simulink model "BCM_C1A_CombiSwitch_9"  (R2018b)
settings: Solver=FixedStepDiscrete  StartTime=0.0  StopTime=10.0  FixedStep=0.01  RelTol=1e-3
undefined symbols (not defined in the file or in its folder): TYP_CSW_INT_POSITION, TYP_EXT_LIGHTS, TYP_FRONT_WIPER, TYP_LIGHTING_CSW, TYP_REAR_WIPER, TYP_VEHICLE_STATE
libraries: Renault_Library x80, library_BCM x2
(part 2 of 3)

== system BCM_C1A_CombiSwitch_9/CombiSwitch/COMBINATION_SWITCH_FNS/EXTERNAL_LIGHTS_MANAGEMENT ==
  R_EXT_LIGHTS : Inport  OutDataTypeStr=Enum: TYP_EXT_LIGHTS
      settings: AttributesFormatString=Type : %<OutDataTypeStr>
  COMBI_SW_FAILURE_TFAIL : Inport  Port=2  OutDataTypeStr=boolean
      settings: AttributesFormatString=Type : %<OutDataTypeStr>
  LIGHTING_CSW_FAILURE_MODE : Inport  Port=3  OutDataTypeStr=boolean
      settings: AttributesFormatString=Type : %<OutDataTypeStr>
  CSW_IN_FAILURE_MODE : Inport  Port=4  OutDataTypeStr=boolean
      settings: AttributesFormatString=Type : %<OutDataTypeStr>
  IN_DRIVING_CYCLE : Inport  Port=5  OutDataTypeStr=boolean
      settings: AttributesFormatString=Type : %<OutDataTypeStr>
  LIGHTING_CSW_CONFIGURATION_CF : Inport  Port=6  OutDataTypeStr=Enum: TYP_LIGHTING_CSW
      settings: AttributesFormatString=Type : %<OutDataTypeStr>
  Constant1 : Constant  Value=TYP_LIGHTING_CSW.LIGHTING_CSW_WORLD_WITHOUT_ALS  OutDataTypeStr=Enum: TYP_LIGHTING_CSW  SampleTime=-1
  Constant2 : Constant  Value=TYP_LIGHTING_CSW.LIGHTING_CSW_WORLD_WITH_ALS  OutDataTypeStr=Enum: TYP_LIGHTING_CSW  SampleTime=-1
  Constant4 : Constant  Value=TYP_LIGHTING_CSW.LIGHTING_CSW_FOR_EUROPE  OutDataTypeStr=Enum: TYP_LIGHTING_CSW  SampleTime=-1
  Constant5 : Constant  Value=TYP_LIGHTING_CSW.LIGHTING_CSW_FOR_EUROPE  OutDataTypeStr=Enum: TYP_LIGHTING_CSW  SampleTime=-1
  LogicalOperator : Logic  Operator=OR  OutDataTypeStr=boolean
  R_LIGHT_SW_EUROPE : Subsystem  TreatAsAtomicUnit=on
      settings: RTWSystemCode=Inline
  R_LIGHT_SW_WORLD : Subsystem  TreatAsAtomicUnit=on
      settings: RTWSystemCode=Inline
  RelationalOperator{,1..3} (4 alike) : RelationalOperator  Operator===  OutDataTypeStr=boolean  RndMeth=Nearest  InputSameDT=on
  Switch : Switch  Criteria=u2 ~= 0  RndMeth=Zero  InputSameDT=on
      settings: AttributesFormatString=Criteria=%<Criteria>
  R_LIGHTS_SW : Outport  OutDataTypeStr=Enum: TYP_EXT_LIGHTS
      settings: AttributesFormatString=Type : %<OutDataTypeStr>\nInit :%<InitialOutput>
  wires:
  [IN_DRIVING_CYCLE] -> R_LIGHT_SW_WORLD/5(IN_DRIVING_CYCLE)
  [LIGHTING_CSW_FAILURE_MODE] -> R_LIGHT_SW_WORLD/3(LIGHTING_CSW_FAILURE_MODE)
  [COMBI_SW_FAILURE_TFAIL] -> R_LIGHT_SW_WORLD/2(COMBI_SW_FAILURE_TFAIL)
  [CSW_IN_FAILURE_MODE] -> R_LIGHT_SW_WORLD/4(CSW_IN_FAILURE_MODE)
  [R_EXT_LIGHTS] -> R_LIGHT_SW_WORLD/1(R_EXT_LIGHTS)
  LIGHTING_CSW_CONFIGURATION_CF/1 -> [LIGHTING_CSW_CONFIGURATION_CF]
  R_EXT_LIGHTS/1 -> [R_EXT_LIGHTS]
  IN_DRIVING_CYCLE/1 -> [IN_DRIVING_CYCLE]
  CSW_IN_FAILURE_MODE/1 -> [CSW_IN_FAILURE_MODE]
  LIGHTING_CSW_FAILURE_MODE/1 -> [LIGHTING_CSW_FAILURE_MODE]
  COMBI_SW_FAILURE_TFAIL/1 -> [COMBI_SW_FAILURE_TFAIL]
  [IN_DRIVING_CYCLE] -> R_LIGHT_SW_EUROPE/5(IN_DRIVING_CYCLE)
  [LIGHTING_CSW_FAILURE_MODE] -> R_LIGHT_SW_EUROPE/3(LIGHTING_CSW_FAILURE_MODE)
  [COMBI_SW_FAILURE_TFAIL] -> R_LIGHT_SW_EUROPE/2(COMBI_SW_FAILURE_TFAIL)
  [CSW_IN_FAILURE_MODE] -> R_LIGHT_SW_EUROPE/4(CSW_IN_FAILURE_MODE)
  [R_EXT_LIGHTS] -> R_LIGHT_SW_EUROPE/1(R_EXT_LIGHTS)
  RelationalOperator1/1 -> R_LIGHT_SW_EUROPE/Enable
  [LIGHTING_CSW_CONFIGURATION_CF] -> RelationalOperator1/1
  [LIGHTING_CSW_CONFIGURATION_CF] -> RelationalOperator/1
  Constant2/1 -> RelationalOperator/2
  Constant1/1 -> RelationalOperator2/2
  [LIGHTING_CSW_CONFIGURATION_CF] -> RelationalOperator2/1
  RelationalOperator/1 -> LogicalOperator/1
  RelationalOperator2/1 -> LogicalOperator/2
  LogicalOperator/1 -> R_LIGHT_SW_WORLD/Enable
  [LIGHTING_CSW_CONFIGURATION_CF] -> RelationalOperator3/1
  Constant5/1 -> RelationalOperator3/2
  RelationalOperator3/1 -> Switch/2
  Switch/1 -> R_LIGHTS_SW/1
  R_LIGHT_SW_EUROPE/1(R_LIGHTS_SW_EUROPE) -> Switch/1
  R_LIGHT_SW_WORLD/1(R_LIGHTS_SW_WORLD) -> Switch/3
  Constant4/1 -> RelationalOperator1/2

== system BCM_C1A_CombiSwitch_9/CombiSwitch/COMBINATION_SWITCH_FNS/FLASHERS_MANAGEMENT ==
  R_FLASH_LEFT : Inport  OutDataTypeStr=boolean
      settings: AttributesFormatString=Type : %<OutDataTypeStr>
  R_FLASH_RIGHT : Inport  Port=2  OutDataTypeStr=boolean
      settings: AttributesFormatString=Type : %<OutDataTypeStr>
  R_FLASH_LEFT_SW : Outport  OutDataTypeStr=boolean
      settings: AttributesFormatString=Type : %<OutDataTypeStr>\nInit :%<InitialOutput>
  R_FLASH_RIGHT_SW : Outport  Port=2  OutDataTypeStr=boolean
      settings: AttributesFormatString=Type : %<OutDataTypeStr>\nInit :%<InitialOutput>
  wires:
  R_FLASH_RIGHT/1 -> R_FLASH_RIGHT_SW/1
  R_FLASH_LEFT/1 -> R_FLASH_LEFT_SW/1

== system BCM_C1A_CombiSwitch_9/CombiSwitch/COMBINATION_SWITCH_FNS/FRONT_FOG_MANAGEMENT ==
  R_FR_FOG : Inport  OutDataTypeStr=boolean
      settings: AttributesFormatString=Type : %<OutDataTypeStr>
  COMBI_SW_FAILURE_TFAIL : Inport  Port=2  OutDataTypeStr=boolean
      settings: AttributesFormatString=Type : %<OutDataTypeStr>
  LogicalOperator : Logic  OutDataTypeStr=boolean
  LogicalOperator1 : Logic  Operator=NOT  Inputs=1  OutDataTypeStr=boolean
  R_FR_FOG_SW : Outport  OutDataTypeStr=boolean
      settings: AttributesFormatString=Type : %<OutDataTypeStr>\nInit :%<InitialOutput>
  wires:
  R_FR_FOG/1 -> LogicalOperator/1
  LogicalOperator1/1 -> LogicalOperator/2
  LogicalOperator/1 -> R_FR_FOG_SW/1
  COMBI_SW_FAILURE_TFAIL/1 -> LogicalOperator1/1

== system BCM_C1A_CombiSwitch_9/CombiSwitch/COMBINATION_SWITCH_FNS/FRONT_WIPER_MANAGEMENT ==
  R_FRONT_WIPER : Inport  OutDataTypeStr=Enum: TYP_FRONT_WIPER
      settings: AttributesFormatString=Type : %<OutDataTypeStr>
  R_INT_TIME : Inport  Port=2  OutDataTypeStr=Enum: TYP_CSW_INT_POSITION
      settings: AttributesFormatString=Type : %<OutDataTypeStr>
  CSW_IN_FAILURE_MODE : Inport  Port=3  OutDataTypeStr=boolean
      settings: AttributesFormatString=Type : %<OutDataTypeStr>
  COMBI_SW_FAILURE_TFAIL : Inport  Port=4  OutDataTypeStr=boolean
      settings: AttributesFormatString=Type : %<OutDataTypeStr>
  IN_DRIVING_CYCLE : Inport  Port=5  OutDataTypeStr=boolean
      settings: AttributesFormatString=Type : %<OutDataTypeStr>
  Constant1 : Constant  Value=TYP_FRONT_WIPER.CSW_OFF_FW  OutDataTypeStr=Enum: TYP_FRONT_WIPER  SampleTime=-1
  LogicalOperator2 : Logic  Operator=OR  OutDataTypeStr=boolean
  LogicalOperator3 : Logic  OutDataTypeStr=boolean
  LogicalOperator4 : Logic  Operator=NOT  Inputs=1  OutDataTypeStr=boolean
  LogicalOperator6 : Logic  OutDataTypeStr=boolean
  RSA_DetectChange_v01_04 : Renault_Library/Complex blocks/Logic & Bit Operations/RSA_DetectChange_v01_04  Tag=[LIB]  chkini=on  vinit=false
      settings: AttributesFormatString=%<MaskType> : Ver : 01.04\nCompare the Input with Initial Value = %<chkini>\nInitial Value : = %<vinit>
  RSA_DetectChange_v01_1 : Renault_Library/Complex blocks/Logic & Bit Operations/RSA_DetectChange_v01_04  Tag=[LIB]  chkini=on  vinit=false
      settings: AttributesFormatString=%<MaskType> : Ver : 01.04\nCompare the Input with Initial Value = %<chkini>\nInitial Value : = %<vinit>
  Switch1 : Switch  Criteria=u2 ~= 0  RndMeth=Zero  InputSameDT=on
      settings: AttributesFormatString=Criteria=%<Criteria>
  Switch4 : Switch  Criteria=u2 ~= 0  RndMeth=Zero  InputSameDT=on
      settings: AttributesFormatString=Criteria=%<Criteria>
  Switch6 : Switch  Criteria=u2 ~= 0  RndMeth=Zero  InputSameDT=on
      settings: AttributesFormatString=Criteria=%<Criteria>
  UnitDelay : UnitDelay  InitialCondition=TYP_FRONT_WIPER.CSW_OFF_FW  SampleTime=-1
      settings: AttributesFormatString=IC = %<X0>
  UnitDelay2 : UnitDelay  InitialCondition=TYP_CSW_INT_POSITION.CSW_INTERMITTENT_POSITION_1  SampleTime=-1
      settings: AttributesFormatString=IC = %<X0>
  R_FR_WIPER_SW : Outport  OutDataTypeStr=Enum: TYP_FRONT_WIPER
      settings: AttributesFormatString=Type : %<OutDataTypeStr>\nInit :%<InitialOutput>
  R_INT_SW : Outport  Port=2  OutDataTypeStr=Enum: TYP_CSW_INT_POSITION
      settings: AttributesFormatString=Type : %<OutDataTypeStr>\nInit :%<InitialOutput>
  wires:
  [R_INT_TIME] -> Switch6/3
  R_INT_TIME/1 -> [R_INT_TIME]
  [R_FRONT_WIPER] -> Switch4/3
  R_FRONT_WIPER/1 -> [R_FRONT_WIPER]
  RSA_DetectChange_v01_1/1 -> LogicalOperator2/2
  RSA_DetectChange_v01_04/1 -> LogicalOperator2/1
  LogicalOperator4/1 -> LogicalOperator6/2
  LogicalOperator3/1 -> Switch1/2
  LogicalOperator6/1 -> LogicalOperator3/2
  LogicalOperator2/1 -> LogicalOperator3/1
  [IN_DRIVING_CYCLE] -> RSA_DetectChange_v01_1/1
  [CSW_IN_FAILURE_MODE] -> RSA_DetectChange_v01_04/1
  UnitDelay2/1 -> Switch6/1
  [COMBI_SW_FAILURE_TFAIL] -> Switch6/2
  [R_INT_SW] -> UnitDelay2/1
  Switch1/1 -> Switch4/1
  [COMBI_SW_FAILURE_TFAIL] -> Switch4/2
  Switch6/1 -> R_INT_SW/1, [R_INT_SW]
  [IN_DRIVING_CYCLE] -> LogicalOperator4/1
  UnitDelay/1 -> Switch1/3
  [R_FR_WIPER_SW] -> UnitDelay/1
  Constant1/1 -> Switch1/1
  Switch4/1 -> [R_FR_WIPER_SW], R_FR_WIPER_SW/1
  [CSW_IN_FAILURE_MODE] -> LogicalOperator6/1
  CSW_IN_FAILURE_MODE/1 -> [CSW_IN_FAILURE_MODE]
  COMBI_SW_FAILURE_TFAIL/1 -> [COMBI_SW_FAILURE_TFAIL]
  IN_DRIVING_CYCLE/1 -> [IN_DRIVING_CYCLE]

== system BCM_C1A_CombiSwitch_9/CombiSwitch/COMBINATION_SWITCH_FNS/HIGH_BEAM_MANAGEMENT ==
  R_HIGH_BEAM : Inport  OutDataTypeStr=boolean
      settings: AttributesFormatString=Type : %<OutDataTypeStr>
  LIGHTING_CSW_FAILURE_MODE : Inport  Port=2  OutDataTypeStr=boolean
      settings: AttributesFormatString=Type : %<OutDataTypeStr>
  CSW_IN_FAILURE_MODE : Inport  Port=3  OutDataTypeStr=boolean
      settings: AttributesFormatString=Type : %<OutDataTypeStr>
  LogicalOperator1 : Logic  Operator=OR  OutDataTypeStr=boolean
  LogicalOperator13 : Logic  Operator=NOT  Inputs=1  OutDataTypeStr=boolean
  LogicalOperator14 : Logic  OutDataTypeStr=boolean
  R_HI_BEAM_SW : Outport  OutDataTypeStr=boolean
      settings: AttributesFormatString=Type : %<OutDataTypeStr>\nInit :%<InitialOutput>
  wires:
  [R_HIGH_BEAM] -> LogicalOperator14/2
  R_HIGH_BEAM/1 -> [R_HIGH_BEAM]
  LogicalOperator14/1 -> R_HI_BEAM_SW/1
  [CSW_IN_FAILURE_MODE] -> LogicalOperator1/1
  LogicalOperator1/1 -> LogicalOperator13/1
  [LIGHTING_CSW_FAILURE_MODE] -> LogicalOperator1/2
  CSW_IN_FAILURE_MODE/1 -> [CSW_IN_FAILURE_MODE]
  LIGHTING_CSW_FAILURE_MODE/1 -> [LIGHTING_CSW_FAILURE_MODE]
  LogicalOperator13/1 -> LogicalOperator14/1

== system BCM_C1A_CombiSwitch_9/CombiSwitch/COMBINATION_SWITCH_FNS/MMI ==
  R_FR_FOG_SW : Inport  OutDataTypeStr=boolean
      settings: AttributesFormatString=Type : %<OutDataTypeStr>
  R_RR_FOG_SW : Inport  Port=2  OutDataTypeStr=boolean
      settings: AttributesFormatString=Type : %<OutDataTypeStr>
  R_PASSING_SW : Inport  Port=3  OutDataTypeStr=boolean
      settings: AttributesFormatString=Type : %<OutDataTypeStr>
  R_FR_WASHER_SW : Inport  Port=4  OutDataTypeStr=boolean
      settings: AttributesFormatString=Type : %<OutDataTypeStr>
  R_RR_WASHER_SW : Inport  Port=5  OutDataTypeStr=boolean
      settings: AttributesFormatString=Type : %<OutDataTypeStr>
  R_FLASH_LEFT_SW : Inport  Port=6  OutDataTypeStr=boolean
      settings: AttributesFormatString=Type : %<OutDataTypeStr>
  R_FLASH_RIGHT_SW : Inport  Port=7  OutDataTypeStr=boolean
      settings: AttributesFormatString=Type : %<OutDataTypeStr>
  R_HI_BEAM_SW : Inport  Port=8  OutDataTypeStr=boolean
      settings: AttributesFormatString=Type : %<OutDataTypeStr>
  R_LIGHTS_SW : Inport  Port=9  OutDataTypeStr=Enum: TYP_EXT_LIGHTS
      settings: AttributesFormatString=Type : %<OutDataTypeStr>
  R_FR_WIPER_SW : Inport  Port=10  OutDataTypeStr=Enum: TYP_FRONT_WIPER
      settings: AttributesFormatString=Type : %<OutDataTypeStr>
  R_RR_WIPER_SW : Inport  Port=11  OutDataTypeStr=Enum: TYP_REAR_WIPER
      settings: AttributesFormatString=Type : %<OutDataTypeStr>
  DataTypeConversion : DataTypeConversion  OutDataTypeStr=uint8  RndMeth=Zero
      settings: AttributesFormatString=Saturation:%<SaturateOnIntegerOverflow>
  DataTypeConversion1 : DataTypeConversion  OutDataTypeStr=uint8  RndMeth=Zero
      settings: AttributesFormatString=Saturation:%<SaturateOnIntegerOverflow>
  DataTypeConversion2 : DataTypeConversion  OutDataTypeStr=uint8  RndMeth=Zero
      settings: AttributesFormatString=Saturation:%<SaturateOnIntegerOverflow>
  LogicalOperator9 : Logic  Operator=OR  Inputs=11  OutDataTypeStr=boolean
  RSA_DetectChange_v01_04 : Renault_Library/Complex blocks/Logic & Bit Operations/RSA_DetectChange_v01_04  Tag=[LIB]  chkini=off  vinit=false
      settings: AttributesFormatString=%<MaskType> : Ver : 01.04\nCompare the Input with Initial Value = %<chkini>\nInitial Value : = %<vinit>
  RSA_DetectChange_v01_{1..8,10} (9 alike) : Renault_Library/Complex blocks/Logic & Bit Operations/RSA_DetectChange_v01_04  Tag=[LIB]  chkini=off  vinit=false
      settings: AttributesFormatString=%<MaskType> : Ver : 01.04\nCompare the Input with Initial Value = %<chkini>\nInitial Value : = %<vinit>
  RSA_DetectChange_v01_9 : Renault_Library/Complex blocks/Logic & Bit Operations/RSA_DetectChange_v01_04  Tag=[LIB]  chkini=on  vinit=false
      settings: AttributesFormatString=%<MaskType> : Ver : 01.04\nCompare the Input with Initial Value = %<chkini>\nInitial Value : = %<vinit>
  CUSTOMER_ACTION_ON_COMBI_SWITCH : Outport  OutDataTypeStr=boolean
      settings: AttributesFormatString=Type : %<OutDataTypeStr>\nInit :%<InitialOutput>
  wires:
  LogicalOperator9/1 -> CUSTOMER_ACTION_ON_COMBI_SWITCH/1
  DataTypeConversion2/1 -> RSA_DetectChange_v01_7/1
  DataTypeConversion1/1 -> RSA_DetectChange_v01_9/1
  DataTypeConversion/1 -> RSA_DetectChange_v01_10/1
  R_RR_WIPER_SW/1 -> DataTypeConversion/1
  R_FR_WIPER_SW/1 -> DataTypeConversion1/1
  R_HI_BEAM_SW/1 -> RSA_DetectChange_v01_8/1
  R_LIGHTS_SW/1 -> DataTypeConversion2/1
  R_FLASH_LEFT_SW/1 -> RSA_DetectChange_v01_5/1
  R_FLASH_RIGHT_SW/1 -> RSA_DetectChange_v01_6/1
  R_FR_WASHER_SW/1 -> RSA_DetectChange_v01_3/1
  R_RR_WASHER_SW/1 -> RSA_DetectChange_v01_4/1
  R_PASSING_SW/1 -> RSA_DetectChange_v01_2/1
  R_RR_FOG_SW/1 -> RSA_DetectChange_v01_1/1
  R_FR_FOG_SW/1 -> RSA_DetectChange_v01_04/1
  RSA_DetectChange_v01_04/1 -> LogicalOperator9/1
  RSA_DetectChange_v01_1/1 -> LogicalOperator9/2
  RSA_DetectChange_v01_2/1 -> LogicalOperator9/3
  RSA_DetectChange_v01_3/1 -> LogicalOperator9/4
  RSA_DetectChange_v01_4/1 -> LogicalOperator9/5
  RSA_DetectChange_v01_5/1 -> LogicalOperator9/6
  RSA_DetectChange_v01_6/1 -> LogicalOperator9/7
  RSA_DetectChange_v01_7/1 -> LogicalOperator9/8
  RSA_DetectChange_v01_8/1 -> LogicalOperator9/9
  RSA_DetectChange_v01_9/1 -> LogicalOperator9/10
  RSA_DetectChange_v01_10/1 -> LogicalOperator9/11

== system BCM_C1A_CombiSwitch_9/CombiSwitch/COMBINATION_SWITCH_FNS/PASSING_MANAGEMENT ==
  R_PASSING : Inport  OutDataTypeStr=boolean
      settings: AttributesFormatString=Type : %<OutDataTypeStr>
  COMBI_SW_FAILURE_TFAIL : Inport  Port=2  OutDataTypeStr=boolean
      settings: AttributesFormatString=Type : %<OutDataTypeStr>
  LogicalOperator : Logic  OutDataTypeStr=boolean
  LogicalOperator1 : Logic  Operator=NOT  Inputs=1  OutDataTypeStr=boolean
  R_PASSING_SW : Outport  OutDataTypeStr=boolean
      settings: AttributesFormatString=Type : %<OutDataTypeStr>\nInit :%<InitialOutput>
  wires:
  LogicalOperator/1 -> R_PASSING_SW/1
  R_PASSING/1 -> LogicalOperator/1
  LogicalOperator1/1 -> LogicalOperator/2
  COMBI_SW_FAILURE_TFAIL/1 -> LogicalOperator1/1

== system BCM_C1A_CombiSwitch_9/CombiSwitch/COMBINATION_SWITCH_FNS/REAR_FOG_MANAGEMENT ==
  R_RR_FOG : Inport  OutDataTypeStr=boolean
      settings: AttributesFormatString=Type : %<OutDataTypeStr>
  COMBI_SW_FAILURE_TFAIL : Inport  Port=2  OutDataTypeStr=boolean
      settings: AttributesFormatString=Type : %<OutDataTypeStr>
  LogicalOperator : Logic  OutDataTypeStr=boolean
  LogicalOperator1 : Logic  Operator=NOT  Inputs=1  OutDataTypeStr=boolean
  R_RR_FOG_SW : Outport  OutDataTypeStr=boolean
      settings: AttributesFormatString=Type : %<OutDataTypeStr>\nInit :%<InitialOutput>
  wires:
  R_RR_FOG/1 -> LogicalOperator/1
  LogicalOperator1/1 -> LogicalOperator/2
  LogicalOperator/1 -> R_RR_FOG_SW/1
  COMBI_SW_FAILURE_TFAIL/1 -> LogicalOperator1/1

== system BCM_C1A_CombiSwitch_9/CombiSwitch/COMBINATION_SWITCH_FNS/REAR_WIPER_MANAGEMENT ==
  R_RR_WIPER : Inport  OutDataTypeStr=Enum: TYP_REAR_WIPER
      settings: AttributesFormatString=Type : %<OutDataTypeStr>
  COMBI_SW_FAILURE_TFAIL : Inport  Port=2  OutDataTypeStr=boolean
      settings: AttributesFormatString=Type : %<OutDataTypeStr>
  CSW_IN_FAILURE_MODE : Inport  Port=3  OutDataTypeStr=boolean
      settings: AttributesFormatString=Type : %<OutDataTypeStr>
  IN_DRIVING_CYCLE : Inport  Port=4  OutDataTypeStr=boolean
      settings: AttributesFormatString=Type : %<OutDataTypeStr>
  Constant1 : Constant  Value=TYP_REAR_WIPER.CSW_NO_RR_WIPE  OutDataTypeStr=Enum: TYP_REAR_WIPER  SampleTime=-1
  LogicalOperator2 : Logic  OutDataTypeStr=boolean
  LogicalOperator3 : Logic  Operator=NOT  Inputs=1  OutDataTypeStr=boolean
  RSA_DetectIncrease_v01_04 : Renault_Library/Complex blocks/Logic & Bit Operations/RSA_DetectIncrease_v01_04  Tag=[LIB]  chkini=on  vinit=false
      settings: AttributesFormatString=%<MaskType> : Ver : 01.04\nCompare the Input with Initial Value = %<chkini>\nInitial Value : = %<vinit>
  Switch : Switch  Criteria=u2 ~= 0  RndMeth=Zero  InputSameDT=on
      settings: AttributesFormatString=Criteria=%<Criteria>
  Switch1 : Switch  Criteria=u2 ~= 0  RndMeth=Zero  InputSameDT=on
      settings: AttributesFormatString=Criteria=%<Criteria>
  UnitDelay : UnitDelay  InitialCondition=TYP_REAR_WIPER.CSW_NO_RR_WIPE  SampleTime=-1
      settings: AttributesFormatString=IC = %<X0>
  R_RR_WIPER_SW : Outport  OutDataTypeStr=Enum: TYP_REAR_WIPER
      settings: AttributesFormatString=Type : %<OutDataTypeStr>\nInit :%<InitialOutput>
  wires:
  RSA_DetectIncrease_v01_04/1 -> Switch1/2
  Switch1/1 -> Switch/1
  R_RR_WIPER/1 -> Switch/3
  LogicalOperator3/1 -> LogicalOperator2/2
  UnitDelay/1 -> Switch1/3
  [R_RR_WIPER_SW] -> UnitDelay/1
  Constant1/1 -> Switch1/1
  LogicalOperator2/1 -> RSA_DetectIncrease_v01_04/1
  CSW_IN_FAILURE_MODE/1 -> LogicalOperator2/1
  IN_DRIVING_CYCLE/1 -> LogicalOperator3/1
  COMBI_SW_FAILURE_TFAIL/1 -> Switch/2
  Switch/1 -> [R_RR_WIPER_SW], R_RR_WIPER_SW/1

== system BCM_C1A_CombiSwitch_9/CombiSwitch/COMBINATION_SWITCH_FNS/WASHERS_MANAGEMENT ==
  R_FR_WASHER : Inport  OutDataTypeStr=boolean
      settings: AttributesFormatString=Type : %<OutDataTypeStr>
  R_RR_WASHER : Inport  Port=2  OutDataTypeStr=boolean
      settings: AttributesFormatString=Type : %<OutDataTypeStr>
  COMBI_SW_FAILURE_TFAIL : Inport  Port=3  OutDataTypeStr=boolean
      settings: AttributesFormatString=Type : %<OutDataTypeStr>
  LogicalOperator : Logic  Inputs=3  OutDataTypeStr=boolean
  LogicalOperator{2..3,6..7} (4 alike) : Logic  Operator=NOT  Inputs=1  OutDataTypeStr=boolean
  LogicalOperator5 : Logic  Inputs=3  OutDataTypeStr=boolean
  R_FR_WASHER_SW : Outport  OutDataTypeStr=boolean
      settings: AttributesFormatString=Type : %<OutDataTypeStr>\nInit :%<InitialOutput>
  R_RR_WASHER_SW : Outport  Port=2  OutDataTypeStr=boolean
      settings: AttributesFormatString=Type : %<OutDataTypeStr>\nInit :%<InitialOutput>
  wires:
  LogicalOperator5/1 -> R_RR_WASHER_SW/1
  LogicalOperator6/1 -> LogicalOperator5/2
  LogicalOperator7/1 -> LogicalOperator5/3
  [COMBI_SW_FAILURE_TFAIL] -> LogicalOperator7/1
  [R_FR_WASHER] -> LogicalOperator6/1
  [R_RR_WASHER] -> LogicalOperator5/1
  LogicalOperator2/1 -> LogicalOperator/2
  LogicalOperator3/1 -> LogicalOperator/3
  [COMBI_SW_FAILURE_TFAIL] -> LogicalOperator3/1
  [R_RR_WASHER] -> LogicalOperator2/1
  [R_FR_WASHER] -> LogicalOperator/1
  LogicalOperator/1 -> R_FR_WASHER_SW/1
  R_FR_WASHER/1 -> [R_FR_WASHER]
  R_RR_WASHER/1 -> [R_RR_WASHER]
  COMBI_SW_FAILURE_TFAIL/1 -> [COMBI_SW_FAILURE_TFAIL]

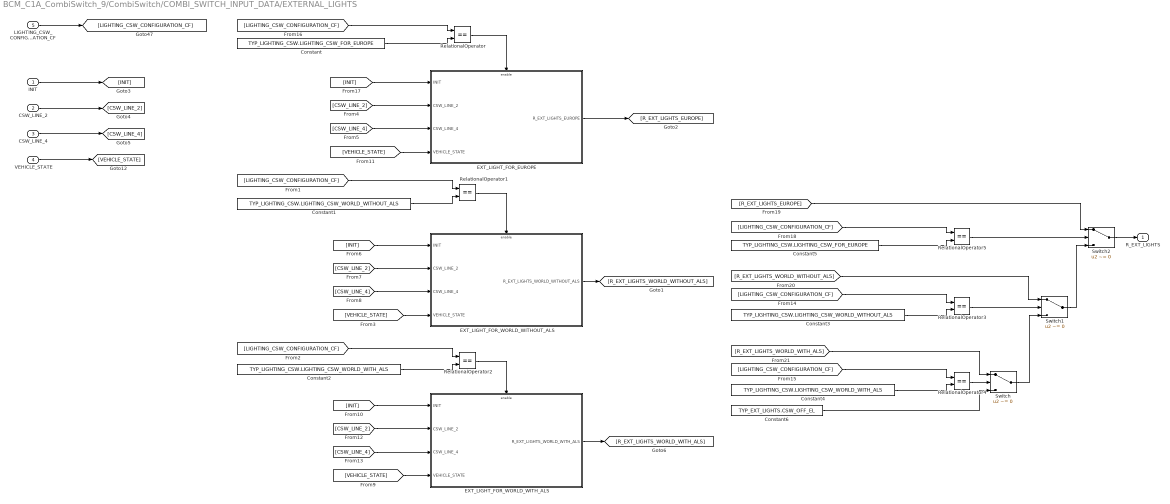
== system BCM_C1A_CombiSwitch_9/CombiSwitch/COMBI_SWITCH_INPUT_DATA/EXTERNAL_LIGHTS ==
  INIT : Inport  OutDataTypeStr=boolean
      settings: AttributesFormatString=Type : %<OutDataTypeStr>
  CSW_LINE_2 : Inport  Port=2  OutDataTypeStr=boolean  PortDimensions=6
      settings: AttributesFormatString=Type : %<OutDataTypeStr>
  CSW_LINE_4 : Inport  Port=3  OutDataTypeStr=boolean  PortDimensions=6
      settings: AttributesFormatString=Type : %<OutDataTypeStr>
  VEHICLE_STATE : Inport  Port=4  OutDataTypeStr=Enum: TYP_VEHICLE_STATE
      settings: AttributesFormatString=Type : %<OutDataTypeStr>
  LIGHTING_CSW_CONFIGURATION_CF : Inport  Port=5  OutDataTypeStr=Enum: TYP_LIGHTING_CSW
      settings: AttributesFormatString=Type : %<OutDataTypeStr>
  Constant : Constant  Value=TYP_LIGHTING_CSW.LIGHTING_CSW_FOR_EUROPE  OutDataTypeStr=Enum: TYP_LIGHTING_CSW  SampleTime=-1
  Constant1 : Constant  Value=TYP_LIGHTING_CSW.LIGHTING_CSW_WORLD_WITHOUT_ALS  OutDataTypeStr=Enum: TYP_LIGHTING_CSW  SampleTime=-1
  Constant2 : Constant  Value=TYP_LIGHTING_CSW.LIGHTING_CSW_WORLD_WITH_ALS  OutDataTypeStr=Enum: TYP_LIGHTING_CSW  SampleTime=-1
  Constant3 : Constant  Value=TYP_LIGHTING_CSW.LIGHTING_CSW_WORLD_WITHOUT_ALS  OutDataTypeStr=Enum: TYP_LIGHTING_CSW  SampleTime=-1
  Constant4 : Constant  Value=TYP_LIGHTING_CSW.LIGHTING_CSW_WORLD_WITH_ALS  OutDataTypeStr=Enum: TYP_LIGHTING_CSW  SampleTime=-1
  Constant5 : Constant  Value=TYP_LIGHTING_CSW.LIGHTING_CSW_FOR_EUROPE  OutDataTypeStr=Enum: TYP_LIGHTING_CSW  SampleTime=-1
  Constant6 : Constant  Value=TYP_EXT_LIGHTS.CSW_OFF_EL  OutDataTypeStr=Enum: TYP_EXT_LIGHTS  SampleTime=-1
  EXT_LIGHT_FOR_EUROPE : Subsystem  TreatAsAtomicUnit=on
      settings: RTWSystemCode=Inline
  EXT_LIGHT_FOR_WORLD_WITHOUT_ALS : Subsystem  TreatAsAtomicUnit=on
      settings: RTWSystemCode=Inline
  EXT_LIGHT_FOR_WORLD_WITH_ALS : Subsystem  TreatAsAtomicUnit=on
      settings: RTWSystemCode=Inline
  RelationalOperator{,1..5} (6 alike) : RelationalOperator  Operator===  OutDataTypeStr=boolean  RndMeth=Nearest  InputSameDT=on
  Switch : Switch  Criteria=u2 ~= 0  RndMeth=Zero  InputSameDT=on
      settings: AttributesFormatString=Criteria=%<Criteria>
  Switch1 : Switch  Criteria=u2 ~= 0  RndMeth=Zero  InputSameDT=on
      settings: AttributesFormatString=Criteria=%<Criteria>
  Switch2 : Switch  Criteria=u2 ~= 0  RndMeth=Zero  InputSameDT=on
      settings: AttributesFormatString=Criteria=%<Criteria>
  R_EXT_LIGHTS : Outport  OutDataTypeStr=Enum: TYP_EXT_LIGHTS
      settings: AttributesFormatString=Type : %<OutDataTypeStr>\nInit :%<InitialOutput>
  wires:
  Constant/1 -> RelationalOperator/2
  RelationalOperator/1 -> EXT_LIGHT_FOR_EUROPE/Enable
  LIGHTING_CSW_CONFIGURATION_CF/1 -> [LIGHTING_CSW_CONFIGURATION_CF]
  [LIGHTING_CSW_CONFIGURATION_CF] -> RelationalOperator/1
  Constant1/1 -> RelationalOperator1/2
  [LIGHTING_CSW_CONFIGURATION_CF] -> RelationalOperator1/1
  Constant2/1 -> RelationalOperator2/2
  [LIGHTING_CSW_CONFIGURATION_CF] -> RelationalOperator2/1
  RelationalOperator1/1 -> EXT_LIGHT_FOR_WORLD_WITHOUT_ALS/Enable
  RelationalOperator2/1 -> EXT_LIGHT_FOR_WORLD_WITH_ALS/Enable
  [VEHICLE_STATE] -> EXT_LIGHT_FOR_EUROPE/4(VEHICLE_STATE)
  [INIT] -> EXT_LIGHT_FOR_EUROPE/1(INIT)
  [CSW_LINE_2] -> EXT_LIGHT_FOR_EUROPE/2(CSW_LINE_2)
  [CSW_LINE_4] -> EXT_LIGHT_FOR_EUROPE/3(CSW_LINE_4)
  [VEHICLE_STATE] -> EXT_LIGHT_FOR_WORLD_WITHOUT_ALS/4(VEHICLE_STATE)
  [CSW_LINE_2] -> EXT_LIGHT_FOR_WORLD_WITHOUT_ALS/2(CSW_LINE_2)
  [CSW_LINE_4] -> EXT_LIGHT_FOR_WORLD_WITHOUT_ALS/3(CSW_LINE_4)
  [INIT] -> EXT_LIGHT_FOR_WORLD_WITHOUT_ALS/1(INIT)
  [VEHICLE_STATE] -> EXT_LIGHT_FOR_WORLD_WITH_ALS/4(VEHICLE_STATE)
  [INIT] -> EXT_LIGHT_FOR_WORLD_WITH_ALS/1(INIT)
  [CSW_LINE_2] -> EXT_LIGHT_FOR_WORLD_WITH_ALS/2(CSW_LINE_2)
  [CSW_LINE_4] -> EXT_LIGHT_FOR_WORLD_WITH_ALS/3(CSW_LINE_4)
  INIT/1 -> [INIT]
  CSW_LINE_2/1 -> [CSW_LINE_2]
  CSW_LINE_4/1 -> [CSW_LINE_4]
  VEHICLE_STATE/1 -> [VEHICLE_STATE]
  Constant3/1 -> RelationalOperator3/2
  [LIGHTING_CSW_CONFIGURATION_CF] -> RelationalOperator3/1
  Constant4/1 -> RelationalOperator4/2
  [LIGHTING_CSW_CONFIGURATION_CF] -> RelationalOperator4/1
  Constant5/1 -> RelationalOperator5/2
  [LIGHTING_CSW_CONFIGURATION_CF] -> RelationalOperator5/1
  EXT_LIGHT_FOR_EUROPE/1(R_EXT_LIGHTS_EUROPE) -> [R_EXT_LIGHTS_EUROPE]
  EXT_LIGHT_FOR_WORLD_WITH_ALS/1(R_EXT_LIGHTS_WORLD_WITH_ALS) -> [R_EXT_LIGHTS_WORLD_WITH_ALS]
  EXT_LIGHT_FOR_WORLD_WITHOUT_ALS/1(R_EXT_LIGHTS_WORLD_WITHOUT_ALS) -> [R_EXT_LIGHTS_WORLD_WITHOUT_ALS]
  RelationalOperator4/1 -> Switch/2
  RelationalOperator3/1 -> Switch1/2
  Switch/1 -> Switch1/3
  [R_EXT_LIGHTS_WORLD_WITH_ALS] -> Switch/1
  [R_EXT_LIGHTS_WORLD_WITHOUT_ALS] -> Switch1/1
  Switch1/1 -> Switch2/3
  RelationalOperator5/1 -> Switch2/2
  [R_EXT_LIGHTS_EUROPE] -> Switch2/1
  Constant6/1 -> Switch/3
  Switch2/1 -> R_EXT_LIGHTS/1

== system BCM_C1A_CombiSwitch_9/CombiSwitch/COMBI_SWITCH_INPUT_DATA/FLASHERS ==
  CSW_LINE_3 : Inport  OutDataTypeStr=boolean  PortDimensions=6
      settings: AttributesFormatString=Type : %<OutDataTypeStr>
  Selector : Selector  IndexMode=Zero-based  InputPortWidth=6  IndexOptions=Index vector (dialog)  Indices=[3]  OutputSizes=1
  Selector1 : Selector  IndexMode=Zero-based  InputPortWidth=6  IndexOptions=Index vector (dialog)  Indices=[4]  OutputSizes=1
  R_FLASH_LEFT : Outport  OutDataTypeStr=boolean
      settings: AttributesFormatString=Type : %<OutDataTypeStr>\nInit :%<InitialOutput>
  R_FLASH_RIGHT : Outport  Port=2  OutDataTypeStr=boolean
      settings: AttributesFormatString=Type : %<OutDataTypeStr>\nInit :%<InitialOutput>
  wires:
  Selector/1 -> R_FLASH_LEFT/1
  [CSW_LINE_3] -> Selector1/1
  Selector1/1 -> R_FLASH_RIGHT/1
  CSW_LINE_3/1 -> [CSW_LINE_3]
  [CSW_LINE_3] -> Selector/1

== system BCM_C1A_CombiSwitch_9/CombiSwitch/COMBI_SWITCH_INPUT_DATA/FOG_LAMP ==
  INIT : Inport  OutDataTypeStr=boolean
      settings: AttributesFormatString=Type : %<OutDataTypeStr>
  CSW_LINE_1 : Inport  Port=2  OutDataTypeStr=boolean  PortDimensions=6
      settings: AttributesFormatString=Type : %<OutDataTypeStr>
  Constant1 : Constant  Value=false  OutDataTypeStr=Inherit: Inherit via back propagation  SampleTime=-1
  Constant4 : Constant  Value=false  OutDataTypeStr=Inherit: Inherit via back propagation  SampleTime=-1
  RSA_DetectChange_v01_04 : Renault_Library/Complex blocks/Logic & Bit Operations/RSA_DetectChange_v01_04  Tag=[LIB]  chkini=on  vinit=false
      settings: AttributesFormatString=%<MaskType> : Ver : 01.04\nCompare the Input with Initial Value = %<chkini>\nInitial Value : = %<vinit>
  RSA_DetectChange_v01_1 : Renault_Library/Complex blocks/Logic & Bit Operations/RSA_DetectChange_v01_04  Tag=[LIB]  chkini=on  vinit=false
      settings: AttributesFormatString=%<MaskType> : Ver : 01.04\nCompare the Input with Initial Value = %<chkini>\nInitial Value : = %<vinit>
  Selector : Selector  IndexMode=Zero-based  InputPortWidth=6  IndexOptions=Index vector (dialog)  Indices=[4]  OutputSizes=1
  Selector1 : Selector  IndexMode=Zero-based  InputPortWidth=6  IndexOptions=Index vector (dialog)  Indices=[3]  OutputSizes=1
  Selector2 : Selector  IndexMode=Zero-based  InputPortWidth=6  IndexOptions=Index vector (dialog)  Indices=[4]  OutputSizes=1
  Selector3 : Selector  IndexMode=Zero-based  InputPortWidth=6  IndexOptions=Index vector (dialog)  Indices=[3]  OutputSizes=1
  Switch{1..4} (4 alike) : Switch  Criteria=u2 ~= 0  RndMeth=Zero  InputSameDT=on
      settings: AttributesFormatString=Criteria=%<Criteria>
  UnitDelay1 : UnitDelay  InitialCondition=false  SampleTime=-1
      settings: AttributesFormatString=IC = %<X0>
  UnitDelay2 : UnitDelay  InitialCondition=false  SampleTime=-1
      settings: AttributesFormatString=IC = %<X0>
  R_FR_FOG : Outport  OutDataTypeStr=boolean
      settings: AttributesFormatString=Type : %<OutDataTypeStr>\nInit :%<InitialOutput>
  R_RR_FOG : Outport  Port=2  OutDataTypeStr=boolean
      settings: AttributesFormatString=Type : %<OutDataTypeStr>\nInit :%<InitialOutput>
  wires:
  [CSW_LINE_1] -> Selector3/1
  [R_RR_FOG] -> R_RR_FOG/1
  [R_RR_FOG] -> UnitDelay1/1
  Constant1/1 -> Switch4/1
  Switch1/1 -> Switch4/3
  Switch4/1 -> [R_RR_FOG]
  [INIT] -> Switch4/2
  Selector3/1 -> Switch1/1
  Selector1/1 -> RSA_DetectChange_v01_1/1
  RSA_DetectChange_v01_1/1 -> Switch1/2
  UnitDelay1/1 -> Switch1/3
  [R_FR_FOG] -> UnitDelay2/1
  [CSW_LINE_1] -> Selector2/1
  [CSW_LINE_1] -> Selector/1
  [R_FR_FOG] -> R_FR_FOG/1
  Constant4/1 -> Switch3/1
  Switch2/1 -> Switch3/3
  Switch3/1 -> [R_FR_FOG]
  [INIT] -> Switch3/2
  Selector2/1 -> Switch2/1
  Selector/1 -> RSA_DetectChange_v01_04/1
  RSA_DetectChange_v01_04/1 -> Switch2/2
  UnitDelay2/1 -> Switch2/3
  INIT/1 -> [INIT]
  [CSW_LINE_1] -> Selector1/1
  CSW_LINE_1/1 -> [CSW_LINE_1]

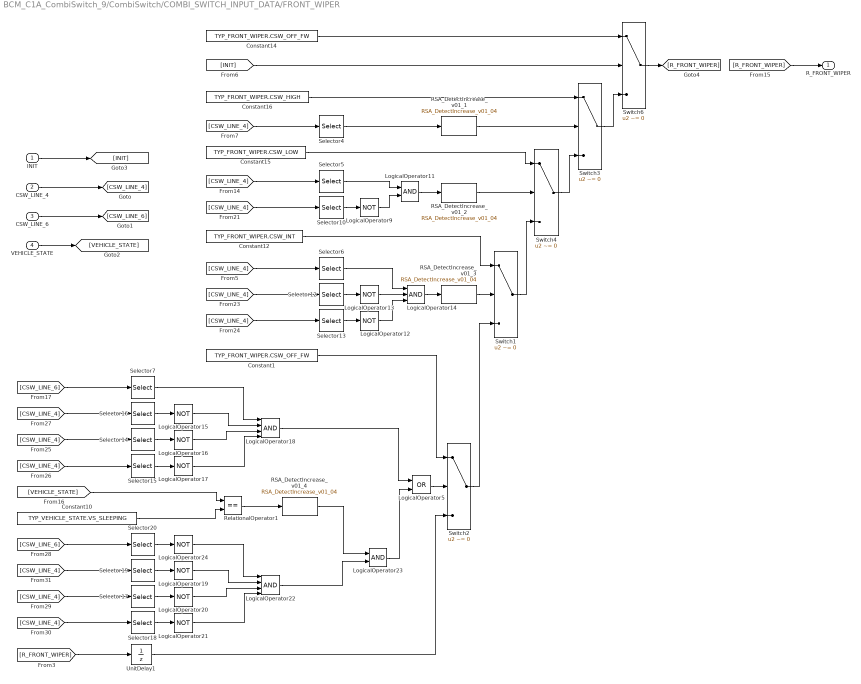
== system BCM_C1A_CombiSwitch_9/CombiSwitch/COMBI_SWITCH_INPUT_DATA/FRONT_WIPER ==
  INIT : Inport  OutDataTypeStr=boolean
      settings: AttributesFormatString=Type : %<OutDataTypeStr>
  CSW_LINE_4 : Inport  Port=2  OutDataTypeStr=boolean  PortDimensions=6
      settings: AttributesFormatString=Type : %<OutDataTypeStr>
  CSW_LINE_6 : Inport  Port=3  OutDataTypeStr=boolean  PortDimensions=6
      settings: AttributesFormatString=Type : %<OutDataTypeStr>
  VEHICLE_STATE : Inport  Port=4  OutDataTypeStr=Enum: TYP_VEHICLE_STATE
      settings: AttributesFormatString=Type : %<OutDataTypeStr>
  Constant1 : Constant  Value=TYP_FRONT_WIPER.CSW_OFF_FW  OutDataTypeStr=Enum: TYP_FRONT_WIPER  SampleTime=-1
  Constant10 : Constant  Value=TYP_VEHICLE_STATE.VS_SLEEPING  OutDataTypeStr=Enum: TYP_VEHICLE_STATE  SampleTime=-1
  Constant12 : Constant  Value=TYP_FRONT_WIPER.CSW_INT  OutDataTypeStr=Enum: TYP_FRONT_WIPER  SampleTime=-1
  Constant14 : Constant  Value=TYP_FRONT_WIPER.CSW_OFF_FW  OutDataTypeStr=Enum: TYP_FRONT_WIPER  SampleTime=-1
  Constant15 : Constant  Value=TYP_FRONT_WIPER.CSW_LOW  OutDataTypeStr=Enum: TYP_FRONT_WIPER  SampleTime=-1
  Constant16 : Constant  Value=TYP_FRONT_WIPER.CSW_HIGH  OutDataTypeStr=Enum: TYP_FRONT_WIPER  SampleTime=-1
  LogicalOperator11 : Logic  OutDataTypeStr=boolean
  LogicalOperator{9,12..13,15..17,19..21,24} (10 alike) : Logic  Operator=NOT  OutDataTypeStr=boolean
  LogicalOperator14 : Logic  Inputs=3  OutDataTypeStr=boolean
  LogicalOperator18 : Logic  Inputs=4  OutDataTypeStr=boolean
  LogicalOperator22 : Logic  Inputs=4  OutDataTypeStr=boolean
  LogicalOperator23 : Logic  OutDataTypeStr=boolean
  LogicalOperator5 : Logic  Operator=OR  OutDataTypeStr=boolean
  RSA_DetectIncrease_v01_{1..4} (4 alike) : Renault_Library/Complex blocks/Logic & Bit Operations/RSA_DetectIncrease_v01_04  Tag=[LIB]  chkini=off  vinit=false
      settings: AttributesFormatString=%<MaskType> : Ver : 01.04\nCompare the Input with Initial Value = %<chkini>\nInitial Value : = %<vinit>
  RelationalOperator1 : RelationalOperator  Operator===  OutDataTypeStr=boolean  RndMeth=Nearest  InputSameDT=on
  Selector{4,10,12,14,17} (5 alike) : Selector  IndexMode=Zero-based  InputPortWidth=6  IndexOptions=Index vector (dialog)  Indices=[1]  OutputSizes=1
  Selector{5,7,13,15,18,20} (6 alike) : Selector  IndexMode=Zero-based  InputPortWidth=6  IndexOptions=Index vector (dialog)  Indices=[0]  OutputSizes=1
  Selector16 : Selector  IndexMode=Zero-based  InputPortWidth=6  IndexOptions=Index vector (dialog)  Indices=[2]  OutputSizes=1
  Selector19 : Selector  IndexMode=Zero-based  InputPortWidth=6  IndexOptions=Index vector (dialog)  Indices=[2]  OutputSizes=1
  Selector6 : Selector  IndexMode=Zero-based  InputPortWidth=6  IndexOptions=Index vector (dialog)  Indices=[2]  OutputSizes=1
  Switch{1..4,6} (5 alike) : Switch  Criteria=u2 ~= 0  RndMeth=Zero  InputSameDT=on
      settings: AttributesFormatString=Criteria=%<Criteria>
  UnitDelay1 : UnitDelay  InitialCondition=TYP_FRONT_WIPER.CSW_OFF_FW  SampleTime=-1
      settings: AttributesFormatString=IC = %<X0>
  R_FRONT_WIPER : Outport  OutDataTypeStr=Enum: TYP_FRONT_WIPER
      settings: AttributesFormatString=Type : %<OutDataTypeStr>\nInit :%<InitialOutput>
  wires:
  VEHICLE_STATE/1 -> [VEHICLE_STATE]
  CSW_LINE_6/1 -> [CSW_LINE_6]
  CSW_LINE_4/1 -> [CSW_LINE_4]
  INIT/1 -> [INIT]
  Switch6/1 -> [R_FRONT_WIPER]
  RelationalOperator1/1 -> RSA_DetectIncrease_v01_4/1
  [INIT] -> Switch6/2
  Constant14/1 -> Switch6/1
  Constant16/1 -> Switch3/1
  Constant15/1 -> Switch4/1
  [R_FRONT_WIPER] -> UnitDelay1/1
  [CSW_LINE_6] -> Selector7/1
  [VEHICLE_STATE] -> RelationalOperator1/1
  Switch1/1 -> Switch4/3
  Switch4/1 -> Switch3/3
  Switch3/1 -> Switch6/3
  Constant12/1 -> Switch1/1
  [CSW_LINE_4] -> Selector4/1
  [CSW_LINE_4] -> Selector5/1
  Selector5/1 -> LogicalOperator11/1
  [CSW_LINE_4] -> Selector6/1
  Selector6/1 -> LogicalOperator14/1
  Selector7/1 -> LogicalOperator18/1
  Constant10/1 -> RelationalOperator1/2
  UnitDelay1/1 -> Switch2/3
  Switch2/1 -> Switch1/3
  Constant1/1 -> Switch2/1
  [R_FRONT_WIPER] -> R_FRONT_WIPER/1
  Selector4/1 -> RSA_DetectIncrease_v01_1/1
  LogicalOperator11/1 -> RSA_DetectIncrease_v01_2/1
  LogicalOperator14/1 -> RSA_DetectIncrease_v01_3/1
  LogicalOperator5/1 -> Switch2/2
  LogicalOperator18/1 -> LogicalOperator5/1
  [CSW_LINE_4] -> Selector10/1
  Selector10/1 -> LogicalOperator9/1
  LogicalOperator9/1 -> LogicalOperator11/2
  [CSW_LINE_4] -> Selector12/1
  [CSW_LINE_4] -> Selector13/1
  Selector12/1 -> LogicalOperator13/1
  Selector13/1 -> LogicalOperator12/1
  LogicalOperator13/1 -> LogicalOperator14/2
  LogicalOperator12/1 -> LogicalOperator14/3
  [CSW_LINE_4] -> Selector16/1
  [CSW_LINE_4] -> Selector14/1
  [CSW_LINE_4] -> Selector15/1
  Selector16/1 -> LogicalOperator15/1
  Selector14/1 -> LogicalOperator16/1
  Selector15/1 -> LogicalOperator17/1
  LogicalOperator17/1 -> LogicalOperator18/4
  LogicalOperator16/1 -> LogicalOperator18/3
  LogicalOperator15/1 -> LogicalOperator18/2
  [CSW_LINE_6] -> Selector20/1
  Selector20/1 -> LogicalOperator24/1
  [CSW_LINE_4] -> Selector19/1
  [CSW_LINE_4] -> Selector17/1
  [CSW_LINE_4] -> Selector18/1
  Selector19/1 -> LogicalOperator19/1
  Selector17/1 -> LogicalOperator20/1
  Selector18/1 -> LogicalOperator21/1
  LogicalOperator21/1 -> LogicalOperator22/4
  LogicalOperator20/1 -> LogicalOperator22/3
  LogicalOperator19/1 -> LogicalOperator22/2
  RSA_DetectIncrease_v01_4/1 -> LogicalOperator23/1
  LogicalOperator23/1 -> LogicalOperator5/2
  LogicalOperator22/1 -> LogicalOperator23/2
  LogicalOperator24/1 -> LogicalOperator22/1
  RSA_DetectIncrease_v01_1/1 -> Switch3/2
  RSA_DetectIncrease_v01_2/1 -> Switch4/2
  RSA_DetectIncrease_v01_3/1 -> Switch1/2

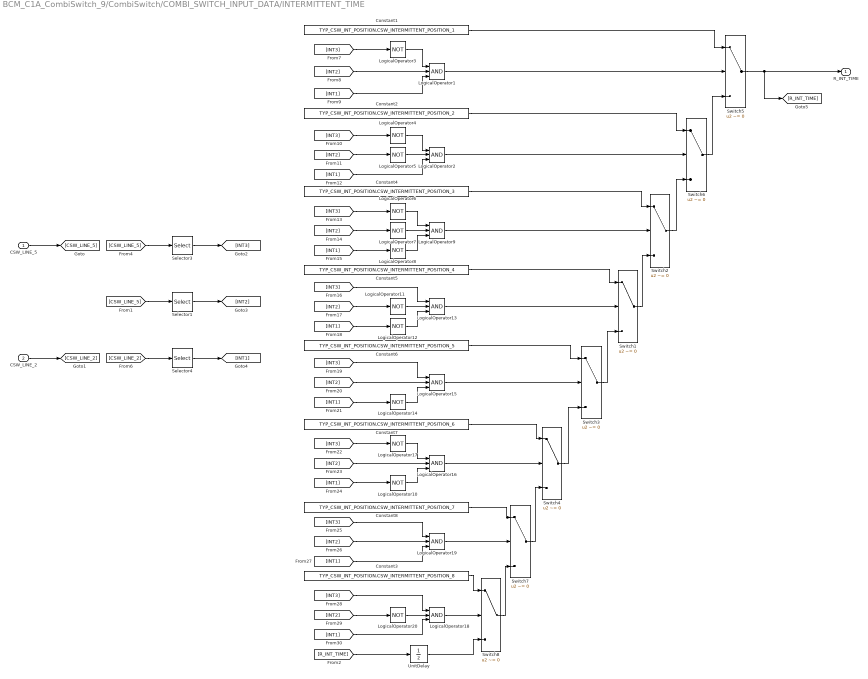
== system BCM_C1A_CombiSwitch_9/CombiSwitch/COMBI_SWITCH_INPUT_DATA/INTERMITTENT_TIME ==
  CSW_LINE_5 : Inport  OutDataTypeStr=boolean  PortDimensions=6
      settings: AttributesFormatString=Type : %<OutDataTypeStr>
  CSW_LINE_2 : Inport  Port=2  OutDataTypeStr=boolean  PortDimensions=6
      settings: AttributesFormatString=Type : %<OutDataTypeStr>
  Constant1 : Constant  Value=TYP_CSW_INT_POSITION.CSW_INTERMITTENT_POSITION_1  OutDataTypeStr=Enum: TYP_CSW_INT_POSITION  SampleTime=-1
  Constant2 : Constant  Value=TYP_CSW_INT_POSITION.CSW_INTERMITTENT_POSITION_2  OutDataTypeStr=Enum: TYP_CSW_INT_POSITION  SampleTime=-1
  Constant3 : Constant  Value=TYP_CSW_INT_POSITION.CSW_INTERMITTENT_POSITION_8  OutDataTypeStr=Enum: TYP_CSW_INT_POSITION  SampleTime=-1
  Constant4 : Constant  Value=TYP_CSW_INT_POSITION.CSW_INTERMITTENT_POSITION_3  OutDataTypeStr=Enum: TYP_CSW_INT_POSITION  SampleTime=-1
  Constant5 : Constant  Value=TYP_CSW_INT_POSITION.CSW_INTERMITTENT_POSITION_4  OutDataTypeStr=Enum: TYP_CSW_INT_POSITION  SampleTime=-1
  Constant6 : Constant  Value=TYP_CSW_INT_POSITION.CSW_INTERMITTENT_POSITION_5  OutDataTypeStr=Enum: TYP_CSW_INT_POSITION  SampleTime=-1
  Constant7 : Constant  Value=TYP_CSW_INT_POSITION.CSW_INTERMITTENT_POSITION_6  OutDataTypeStr=Enum: TYP_CSW_INT_POSITION  SampleTime=-1
  Constant8 : Constant  Value=TYP_CSW_INT_POSITION.CSW_INTERMITTENT_POSITION_7  OutDataTypeStr=Enum: TYP_CSW_INT_POSITION  SampleTime=-1
  LogicalOperator{1..2,9,13,15..16,18..19} (8 alike) : Logic  Inputs=3  OutDataTypeStr=boolean
  LogicalOperator{3..8,10..12,14,17,20} (12 alike) : Logic  Operator=NOT  Inputs=1  OutDataTypeStr=boolean
  Selector1 : Selector  IndexMode=Zero-based  InputPortWidth=6  IndexOptions=Index vector (dialog)  Indices=[0]  OutputSizes=1
  Selector3 : Selector  IndexMode=Zero-based  InputPortWidth=6  IndexOptions=Index vector (dialog)  Indices=[1]  OutputSizes=1
  Selector4 : Selector  IndexMode=Zero-based  InputPortWidth=6  IndexOptions=Index vector (dialog)  Indices=[0]  OutputSizes=1
  Switch{1..8} (8 alike) : Switch  Criteria=u2 ~= 0  RndMeth=Zero  InputSameDT=on
      settings: AttributesFormatString=Criteria=%<Criteria>
  UnitDelay : UnitDelay  InitialCondition=TYP_CSW_INT_POSITION.CSW_INTERMITTENT_POSITION_1  SampleTime=-1
      settings: AttributesFormatString=IC = %<X0>
  R_INT_TIME : Outport  OutDataTypeStr=Enum: TYP_CSW_INT_POSITION
      settings: AttributesFormatString=Type : %<OutDataTypeStr>\nInit :%<InitialOutput>
  wires:
  [CSW_LINE_5] -> Selector3/1
  [CSW_LINE_5] -> Selector1/1
  [CSW_LINE_2] -> Selector4/1
  Switch2/1 -> Switch6/3
  Switch6/1 -> Switch5/3
  Switch5/1 -> [R_INT_TIME], R_INT_TIME/1
  CSW_LINE_2/1 -> [CSW_LINE_2]
  CSW_LINE_5/1 -> [CSW_LINE_5]
  Selector3/1 -> [INT3]
  Selector1/1 -> [INT2]
  Selector4/1 -> [INT1]
  [INT2] -> LogicalOperator1/2
  [INT3] -> LogicalOperator3/1
  [INT1] -> LogicalOperator1/3
  LogicalOperator3/1 -> LogicalOperator1/1
  [INT2] -> LogicalOperator5/1
  [INT3] -> LogicalOperator4/1
  LogicalOperator5/1 -> LogicalOperator2/2
  LogicalOperator4/1 -> LogicalOperator2/1
  [INT1] -> LogicalOperator2/3
  LogicalOperator7/1 -> LogicalOperator9/2
  LogicalOperator8/1 -> LogicalOperator9/3
  LogicalOperator6/1 -> LogicalOperator9/1
  [INT3] -> LogicalOperator6/1
  [INT2] -> LogicalOperator7/1
  [INT1] -> LogicalOperator8/1
  LogicalOperator11/1 -> LogicalOperator13/2
  LogicalOperator12/1 -> LogicalOperator13/3
  [INT3] -> LogicalOperator13/1
  [INT2] -> LogicalOperator11/1
  [INT1] -> LogicalOperator12/1
  [INT2] -> LogicalOperator15/2
  LogicalOperator14/1 -> LogicalOperator15/3
  [INT3] -> LogicalOperator15/1
  [INT1] -> LogicalOperator14/1
  [INT2] -> LogicalOperator16/2
  LogicalOperator10/1 -> LogicalOperator16/3
  [INT3] -> LogicalOperator17/1
  [INT1] -> LogicalOperator10/1
  LogicalOperator17/1 -> LogicalOperator16/1
  [INT2] -> LogicalOperator19/2
  [INT1] -> LogicalOperator19/3
  [INT3] -> LogicalOperator19/1
  [INT2] -> LogicalOperator20/1
  [INT1] -> LogicalOperator18/3
  [INT3] -> LogicalOperator18/1
  LogicalOperator20/1 -> LogicalOperator18/2
  LogicalOperator1/1 -> Switch5/2
  Constant1/1 -> Switch5/1
  LogicalOperator2/1 -> Switch6/2
  Constant2/1 -> Switch6/1
  Switch1/1 -> Switch2/3
  LogicalOperator9/1 -> Switch2/2
  LogicalOperator13/1 -> Switch1/2
  LogicalOperator15/1 -> Switch3/2
  LogicalOperator16/1 -> Switch4/2
  Switch4/1 -> Switch3/3
  Constant5/1 -> Switch1/1
  Constant6/1 -> Switch3/1
  Switch3/1 -> Switch1/3
  Switch7/1 -> Switch4/3
  LogicalOperator18/1 -> Switch8/2
  Constant3/1 -> Switch8/1
  LogicalOperator19/1 -> Switch7/2
  Constant8/1 -> Switch7/1
  Constant7/1 -> Switch4/1
  Switch8/1 -> Switch7/3
  Constant4/1 -> Switch2/1
  [R_INT_TIME] -> UnitDelay/1
  UnitDelay/1 -> Switch8/3

== system BCM_C1A_CombiSwitch_9/CombiSwitch/COMBI_SWITCH_INPUT_DATA/PASSING_AND_HIGH_BEAM ==
  INIT : Inport  OutDataTypeStr=boolean
      settings: AttributesFormatString=Type : %<OutDataTypeStr>
  CSW_LINE_1 : Inport  Port=2  OutDataTypeStr=boolean  PortDimensions=6
      settings: AttributesFormatString=Type : %<OutDataTypeStr>
  Constant1 : Constant  Value=false  OutDataTypeStr=Inherit: Inherit via back propagation  SampleTime=-1
  Constant2 : Constant  Value=false  OutDataTypeStr=Inherit: Inherit via back propagation  SampleTime=-1
  RSA_DetectChange_v01_1 : Renault_Library/Complex blocks/Logic & Bit Operations/RSA_DetectChange_v01_04  Tag=[LIB]  chkini=on  vinit=false
      settings: AttributesFormatString=%<MaskType> : Ver : 01.04\nCompare the Input with Initial Value = %<chkini>\nInitial Value : = %<vinit>
  RSA_DetectChange_v01_3 : Renault_Library/Complex blocks/Logic & Bit Operations/RSA_DetectChange_v01_04  Tag=[LIB]  chkini=on  vinit=false
      settings: AttributesFormatString=%<MaskType> : Ver : 01.04\nCompare the Input with Initial Value = %<chkini>\nInitial Value : = %<vinit>
  Selector : Selector  IndexMode=Zero-based  InputPortWidth=6  IndexOptions=Index vector (dialog)  Indices=[2]  OutputSizes=1
  Selector1 : Selector  IndexMode=Zero-based  InputPortWidth=6  IndexOptions=Index vector (dialog)  Indices=[1]  OutputSizes=1
  Selector2 : Selector  IndexMode=Zero-based  InputPortWidth=6  IndexOptions=Index vector (dialog)  Indices=[2]  OutputSizes=1
  Selector3 : Selector  IndexMode=Zero-based  InputPortWidth=6  IndexOptions=Index vector (dialog)  Indices=[1]  OutputSizes=1
  Switch{1..4} (4 alike) : Switch  Criteria=u2 ~= 0  RndMeth=Zero  InputSameDT=on
      settings: AttributesFormatString=Criteria=%<Criteria>
  UnitDelay1 : UnitDelay  InitialCondition=false  SampleTime=-1
      settings: AttributesFormatString=IC = %<X0>
  UnitDelay2 : UnitDelay  InitialCondition=false  SampleTime=-1
      settings: AttributesFormatString=IC = %<X0>
  R_HIGH_BEAM : Outport  OutDataTypeStr=boolean
      settings: AttributesFormatString=Type : %<OutDataTypeStr>\nInit :%<InitialOutput>
  R_PASSING : Outport  Port=2  OutDataTypeStr=boolean
      settings: AttributesFormatString=Type : %<OutDataTypeStr>\nInit :%<InitialOutput>
  wires:
  Switch4/1 -> [R_HIGH_BEAM]
  Constant2/1 -> Switch4/1
  Switch1/1 -> Switch4/3
  [INIT] -> Switch4/2
  [R_HIGH_BEAM] -> R_HIGH_BEAM/1
  [R_HIGH_BEAM] -> UnitDelay1/1
  UnitDelay1/1 -> Switch1/3
  Selector3/1 -> Switch1/1
  [CSW_LINE_1] -> Selector3/1
  RSA_DetectChange_v01_1/1 -> Switch1/2
  INIT/1 -> [INIT]
  Constant1/1 -> Switch3/1
  Switch2/1 -> Switch3/3
  Switch3/1 -> [R_PASSING]
  [INIT] -> Switch3/2
  Selector2/1 -> Switch2/1
  Selector/1 -> RSA_DetectChange_v01_3/1
  [CSW_LINE_1] -> Selector/1
  CSW_LINE_1/1 -> [CSW_LINE_1]
  [R_PASSING] -> R_PASSING/1
  [R_PASSING] -> UnitDelay2/1
  RSA_DetectChange_v01_3/1 -> Switch2/2
  UnitDelay2/1 -> Switch2/3
  [CSW_LINE_1] -> Selector2/1
  [CSW_LINE_1] -> Selector1/1
  Selector1/1 -> RSA_DetectChange_v01_1/1

== system BCM_C1A_CombiSwitch_9/CombiSwitch/COMBI_SWITCH_INPUT_DATA/REAR_WIPER ==
  INIT : Inport  OutDataTypeStr=boolean
      settings: AttributesFormatString=Type : %<OutDataTypeStr>
  CSW_LINE_5 : Inport  Port=2  OutDataTypeStr=boolean  PortDimensions=6
      settings: AttributesFormatString=Type : %<OutDataTypeStr>
  Constant10 : Constant  Value=TYP_REAR_WIPER.CSW_RR_WIPE_CONT  OutDataTypeStr=Enum: TYP_REAR_WIPER  SampleTime=-1
  Constant11 : Constant  Value=TYP_REAR_WIPER.CSW_RR_WIPE_INT  OutDataTypeStr=Enum: TYP_REAR_WIPER  SampleTime=-1
  Constant12 : Constant  Value=TYP_REAR_WIPER.CSW_NO_RR_WIPE  OutDataTypeStr=Enum: TYP_REAR_WIPER  SampleTime=-1
  Constant14 : Constant  Value=TYP_REAR_WIPER.CSW_NO_RR_WIPE  OutDataTypeStr=Enum: TYP_REAR_WIPER  SampleTime=-1
  LogicalOperator1 : Logic  OutDataTypeStr=boolean
  LogicalOperator2 : Logic  Operator=NOT  OutDataTypeStr=boolean
  LogicalOperator3 : Logic  OutDataTypeStr=boolean
  LogicalOperator5 : Logic  Operator=NOT  OutDataTypeStr=boolean
  LogicalOperator6 : Logic  Operator=NOT  OutDataTypeStr=boolean
  RSA_DetectIncrease_v01_04 : Renault_Library/Complex blocks/Logic & Bit Operations/RSA_DetectIncrease_v01_04  Tag=[LIB]  chkini=off  vinit=false
      settings: AttributesFormatString=%<MaskType> : Ver : 01.04\nCompare the Input with Initial Value = %<chkini>\nInitial Value : = %<vinit>
  RSA_DetectIncrease_v01_1 : Renault_Library/Complex blocks/Logic & Bit Operations/RSA_DetectIncrease_v01_04  Tag=[LIB]  chkini=off  vinit=false
      settings: AttributesFormatString=%<MaskType> : Ver : 01.04\nCompare the Input with Initial Value = %<chkini>\nInitial Value : = %<vinit>
  Selector1 : Selector  IndexMode=Zero-based  InputPortWidth=6  IndexOptions=Index vector (dialog)  Indices=[2]  OutputSizes=1
  Selector4 : Selector  IndexMode=Zero-based  InputPortWidth=6  IndexOptions=Index vector (dialog)  Indices=[3]  OutputSizes=1
  Selector5 : Selector  IndexMode=Zero-based  InputPortWidth=6  IndexOptions=Index vector (dialog)  Indices=[3]  OutputSizes=1
  Selector6 : Selector  IndexMode=Zero-based  InputPortWidth=6  IndexOptions=Index vector (dialog)  Indices=[2]  OutputSizes=1
  Selector7 : Selector  IndexMode=Zero-based  InputPortWidth=6  IndexOptions=Index vector (dialog)  Indices=[3]  OutputSizes=1
  Switch{1..3,5} (4 alike) : Switch  Criteria=u2 ~= 0  RndMeth=Zero  InputSameDT=on
      settings: AttributesFormatString=Criteria=%<Criteria>
  UnitDelay : UnitDelay  InitialCondition=TYP_REAR_WIPER.CSW_NO_RR_WIPE  SampleTime=-1
      settings: AttributesFormatString=IC = %<X0>
  R_RR_WIPER : Outport  OutDataTypeStr=Enum: TYP_REAR_WIPER
      settings: AttributesFormatString=Type : %<OutDataTypeStr>\nInit :%<InitialOutput>
  wires:
  INIT/1 -> [INIT]
  CSW_LINE_5/1 -> [CSW_LINE_5]
  Constant12/1 -> Switch5/1
  Constant10/1 -> Switch1/1
  Constant11/1 -> Switch2/1
  Switch1/1 -> Switch5/3
  [INIT] -> Switch5/2
  [CSW_LINE_5] -> Selector1/1
  [CSW_LINE_5] -> Selector4/1
  Switch2/1 -> Switch1/3
  Switch5/1 -> [R_RR_WIPER]
  [CSW_LINE_5] -> Selector5/1
  [CSW_LINE_5] -> Selector6/1
  Selector5/1 -> LogicalOperator6/1
  Selector6/1 -> LogicalOperator5/1
  [R_RR_WIPER] -> UnitDelay/1
  Constant14/1 -> Switch3/1
  Switch3/1 -> Switch2/3
  UnitDelay/1 -> Switch3/3
  Selector4/1 -> RSA_DetectIncrease_v01_04/1
  LogicalOperator1/1 -> Switch3/2
  [R_RR_WIPER] -> R_RR_WIPER/1
  [CSW_LINE_5] -> Selector7/1
  Selector7/1 -> LogicalOperator2/1
  LogicalOperator2/1 -> LogicalOperator3/2
  LogicalOperator3/1 -> RSA_DetectIncrease_v01_1/1
  RSA_DetectIncrease_v01_04/1 -> Switch1/2
  Selector1/1 -> LogicalOperator3/1
  RSA_DetectIncrease_v01_1/1 -> Switch2/2
  LogicalOperator5/1 -> LogicalOperator1/2
  LogicalOperator6/1 -> LogicalOperator1/1

== system BCM_C1A_CombiSwitch_9/CombiSwitch/COMBI_SWITCH_INPUT_DATA/WASHERS ==
  INIT : Inport  OutDataTypeStr=boolean
      settings: AttributesFormatString=Type : %<OutDataTypeStr>
  CSW_LINE_3 : Inport  Port=2  OutDataTypeStr=boolean  PortDimensions=6
      settings: AttributesFormatString=Type : %<OutDataTypeStr>
  Constant1 : Constant  Value=false  OutDataTypeStr=Inherit: Inherit via back propagation  SampleTime=-1
  Constant4 : Constant  Value=false  OutDataTypeStr=Inherit: Inherit via back propagation  SampleTime=-1
  RSA_DetectChange_v01_3 : Renault_Library/Complex blocks/Logic & Bit Operations/RSA_DetectChange_v01_04  Tag=[LIB]  chkini=on  vinit=false
      settings: AttributesFormatString=%<MaskType> : Ver : 01.04\nCompare the Input with Initial Value = %<chkini>\nInitial Value : = %<vinit>
  RSA_DetectChange_v01_4 : Renault_Library/Complex blocks/Logic & Bit Operations/RSA_DetectChange_v01_04  Tag=[LIB]  chkini=on  vinit=false
      settings: AttributesFormatString=%<MaskType> : Ver : 01.04\nCompare the Input with Initial Value = %<chkini>\nInitial Value : = %<vinit>
  Selector : Selector  IndexMode=Zero-based  InputPortWidth=6  IndexOptions=Index vector (dialog)  Indices=[0]  OutputSizes=1
  Selector1 : Selector  IndexMode=Zero-based  InputPortWidth=6  IndexOptions=Index vector (dialog)  Indices=[1]  OutputSizes=1
  Selector2 : Selector  IndexMode=Zero-based  InputPortWidth=6  IndexOptions=Index vector (dialog)  Indices=[0]  OutputSizes=1
  Selector3 : Selector  IndexMode=Zero-based  InputPortWidth=6  IndexOptions=Index vector (dialog)  Indices=[1]  OutputSizes=1
  Switch{2..5} (4 alike) : Switch  Criteria=u2 ~= 0  RndMeth=Zero  InputSameDT=on
      settings: AttributesFormatString=Criteria=%<Criteria>
  UnitDelay1 : UnitDelay  InitialCondition=false  SampleTime=-1
      settings: AttributesFormatString=IC = %<X0>
  UnitDelay2 : UnitDelay  InitialCondition=false  SampleTime=-1
      settings: AttributesFormatString=IC = %<X0>
  R_FR_WASHER : Outport  OutDataTypeStr=boolean
      settings: AttributesFormatString=Type : %<OutDataTypeStr>\nInit :%<InitialOutput>
  R_RR_WASHER : Outport  Port=2  OutDataTypeStr=boolean
      settings: AttributesFormatString=Type : %<OutDataTypeStr>\nInit :%<InitialOutput>
  wires:
  [CSW_LINE_3] -> Selector3/1
  [R_RR_WASHER] -> R_RR_WASHER/1
  [R_RR_WASHER] -> UnitDelay1/1
  Constant1/1 -> Switch5/1
  Switch4/1 -> Switch5/3
  Switch5/1 -> [R_RR_WASHER]
  [INIT] -> Switch5/2
  Selector3/1 -> Switch4/1
  Selector1/1 -> RSA_DetectChange_v01_4/1
  RSA_DetectChange_v01_4/1 -> Switch4/2
  UnitDelay1/1 -> Switch4/3
  [CSW_LINE_3] -> Selector2/1
  [R_FR_WASHER] -> R_FR_WASHER/1
  [R_FR_WASHER] -> UnitDelay2/1
  Constant4/1 -> Switch3/1
  Switch2/1 -> Switch3/3
  Switch3/1 -> [R_FR_WASHER]
  [INIT] -> Switch3/2
  Selector2/1 -> Switch2/1
  Selector/1 -> RSA_DetectChange_v01_3/1
  RSA_DetectChange_v01_3/1 -> Switch2/2
  UnitDelay2/1 -> Switch2/3
  INIT/1 -> [INIT]
  [CSW_LINE_3] -> Selector1/1
  CSW_LINE_3/1 -> [CSW_LINE_3]
  [CSW_LINE_3] -> Selector/1
